simulink model "LQR_observer_R2018a"  (R2018b)
settings: Solver=ode45  StartTime=0.0  StopTime=simulation_time  MaxStep=0.01  RelTol=1e-3  EnableMultiTasking=on
values from neighbouring files (symbols this model uses):
  Cprime = sol2.getCprime    [exercise2_LQRandObserver.m]
  L = parameters(2)    [ex1.m]    (also in exercise2_LQRandObserver.m = L_options{exp_id})
  noiseMod = sol2.getNoiseModule    [exercise2_LQRandObserver.m]
  path_to_track = []    [exercise3_DynamicProgramming.m]
  Phi = Md.A    [ex1.m]
  sampling_time = 0.1    [exercise1_Linearization.m]    (also in exercise2_LQRandObserver.m = 0.005; exercise3_DynamicProgramming.m = 0.24)
  x0 = {x0_experiment_1,                  x0_experiment_1,                  x0_experiment_1,                  x0_experiment_1,                  x0_experiment_1}    [ex1.m]    (also in ex3.m = [0, 0, 0, 0, 0]'; exercise1_Linearization.m = x0_experiments{exp_id}; exercise3_DynamicProgramming.m = sol3.getInitialState)
undefined symbols (not defined in the file or in its folder): CMes, CObs, DObs, Gam, KDlqr, x0Obs
settings Model: Creator=ezequiel  LastModifiedBy=arne
settings OptimizationCC: LifeSpan=inf
settings DebuggingCC: AllowSymbolicDim=off  LibraryContextMissingDiagnostic=none  SFUnexpectedBacktrackingDiag=warning  SFNoUnconditionalDefaultTransitionDiag=warning  SFExecutionAtInitializationDiag=none
settings ModelReferenceCC: PropagateSignalLabelsOutOfModel=off
settings SFSimCC: SimUseLocalCustomCode=off
settings RTWCC: RTWUseLocalCustomCode=off
settings CodeAppCC: StateflowObjectComments=on
settings GRTTargetCC: TargetLangStandard=C89/C90 (ANSI)
settings ConfigComp: CovMetricSettings=dw  CovHtmlReporting=on  CovSaveCumulativeToWorkspaceVar=on  CovSaveSingleToWorkspaceVar=on  CovExternalEMLEnable=off

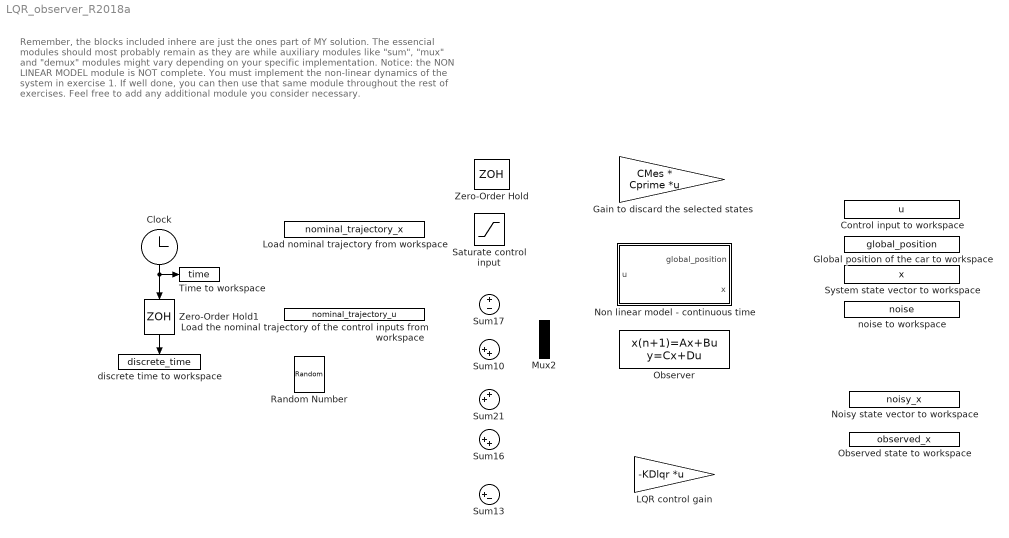
== system LQR_observer_R2018a ==
  note: Remember, the blocks included inhere are just the ones part of MY solution. The essencial modules should most probably remain as they are while auxiliary modules like "sum", "mux" and "demux" modules might vary depending on your specific implementation.
      |
      | Notice: the NON LINEAR MODEL module is NOT complete. You must implement the non-linear dynamics of the system in exercise 1. If well done, you can then use that same module throughout the rest of exercises.
      |
      | Feel free to add any additional module you consider necessary.
  Clock : Clock
  Control input to workspace : ToWorkspace  VariableName=u  SampleTime=-1
  Gain to discard the selected states : Gain  Gain=CMes * Cprime  Multiplication=Matrix(K*u)  SampleTime=sampling_time
  Global position of the car to workspace : ToWorkspace  VariableName=global_position  SampleTime=-1
  LQR control gain : Gain  Gain=-KDlqr  Multiplication=Matrix(K*u)  SampleTime=sampling_time
  Load nominal trajectory from workspace : FromWorkspace  VariableName=nominal_trajectory_x  SampleTime=sampling_time  Interpolate=off  OutputAfterFinalValue=Holding final value
  Load the nominal trajectory of the control inputs from workspace : FromWorkspace  VariableName=nominal_trajectory_u  SampleTime=sampling_time  Interpolate=off  OutputAfterFinalValue=Holding final value
  Mux2 : Mux  Inputs=2
  Noisy state vector to workspace : ToWorkspace  VariableName=noisy_x  SampleTime=-1
  Non linear model - continuous time : Subsystem
  Observed state to workspace : ToWorkspace  VariableName=observed_x  SampleTime=-1
  Observer : DiscreteStateSpace  A=Phi-L*CMes  B=[Gam L]  C=CObs  D=DObs  InitialCondition=x0Obs  SampleTime=sampling_time
  Random Number : RandomNumber  Mean=noiseMod.mean  Variance=noiseMod.std_deviation.^2  Seed=noiseMod.seed  SampleTime=sampling_time
  Saturate control input : Saturate  UpperLimit=[Inf;pi/4]  LowerLimit=[0;-pi/4]
  Sum10 : Sum  Inputs=|++
  Sum13 : Sum  Inputs=|+-
  Sum16 : Sum  Inputs=|++
  Sum17 : Sum  Inputs=+|-
  Sum21 : Sum  Inputs=++|
  System state vector to workspace : ToWorkspace  VariableName=x  SampleTime=-1
  Time to workspace : ToWorkspace  VariableName=time  SampleTime=-1
  Zero-Order Hold : ZeroOrderHold  SampleTime=sampling_time
  Zero-Order Hold1 : ZeroOrderHold  SampleTime=sampling_time
  discrete time to workspace : ToWorkspace  VariableName=discrete_time  SampleTime=-1
  noise to workspace : ToWorkspace  VariableName=noise  SampleTime=-1
  wires:
  Zero-Order Hold1/1 -> discrete time to workspace/1
  Clock/1 -> Zero-Order Hold1/1, Time to workspace/1

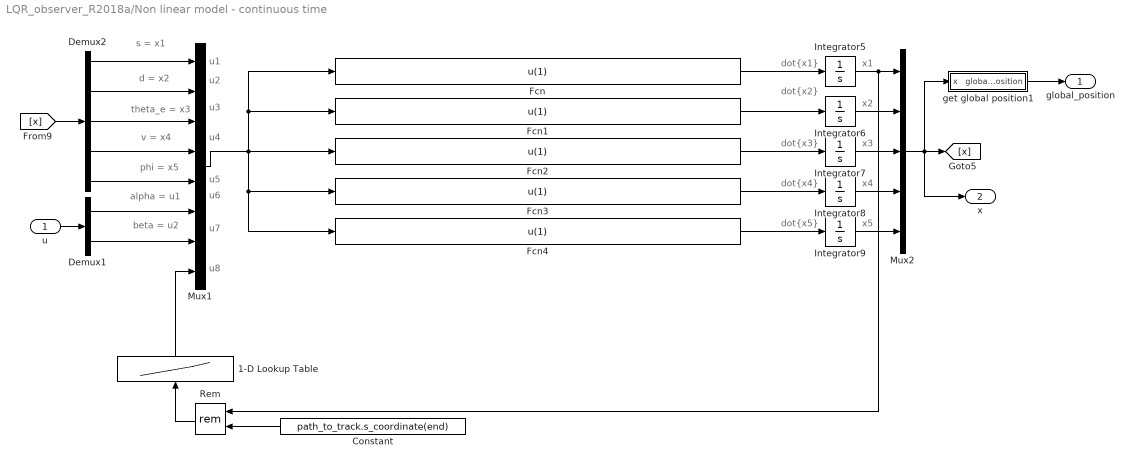
== system LQR_observer_R2018a/Non linear model - continuous time ==
  note: s = x1
  note: dot{x1}
  note: d = x2
  note: theta_e = x3
  note: v = x4
  note: phi = x5
  note: alpha = u1
  note: beta = u2
  note: u1
  note: u2
  note: u3
  note: u4
  note: u5
  note: u6
  note: u7
  note: x1
  note: dot{x2}
  note: x2
  note: dot{x3}
  note: x3
  note: dot{x4}
  note: x4
  note: dot{x5}
  note: x5
  note: u8
  u : Inport
  1-D Lookup Table : Lookup_n-D  NumberOfTableDimensions=1  BreakpointsForDimension1=path_to_track.s_coordinate  Table=path_to_track.curvature  InternalRulePriority=Speed  RndMeth=Simplest  InputSameDT=on
  Constant : Constant  Value=path_to_track.s_coordinate(end)
  Demux1 : Demux  Outputs=2
  Demux2 : Demux  Outputs=5
  Fcn{,1..4} (5 alike) : Fcn  Expr=u(1)
  Integrator5 : Integrator  InitialCondition=x0(1)
  Integrator6 : Integrator  InitialCondition=x0(2)
  Integrator7 : Integrator  InitialCondition=x0(3)
  Integrator8 : Integrator  InitialCondition=x0(4)
  Integrator9 : Integrator  InitialCondition=x0(5)
  Mux1 : Mux  Inputs=8
  Mux2 : Mux  Inputs=5
  Rem : Math  Operator=rem  SaturateOnIntegerOverflow=on
  get global position1 : Subsystem
  global_position : Outport
  x : Outport  Port=2
  wires:
  u/1 -> Demux1/1
  Fcn/1 -> Integrator5/1
  Demux2/1 -> Mux1/1
  Demux2/2 -> Mux1/2
  Demux2/3 -> Mux1/3
  Demux2/4 -> Mux1/4
  Demux2/5 -> Mux1/5
  Demux1/1 -> Mux1/6
  Demux1/2 -> Mux1/7
  Mux1/1 -> Fcn3/1, Fcn4/1, Fcn1/1, Fcn/1, Fcn2/1
  Fcn1/1 -> Integrator6/1
  Integrator6/1 -> Mux2/2
  Fcn2/1 -> Integrator7/1
  Integrator7/1 -> Mux2/3
  Fcn3/1 -> Integrator8/1
  Integrator8/1 -> Mux2/4
  Fcn4/1 -> Integrator9/1
  Integrator9/1 -> Mux2/5
  [x] -> Demux2/1
  1-D Lookup Table/1 -> Mux1/8
  Rem/1 -> 1-D Lookup Table/1
  Constant/1 -> Rem/2
  Integrator5/1 -> Rem/1, Mux2/1
  Mux2/1 -> get global position1/1(x), x/1, [x]
  get global position1/1(global_position) -> global_position/1

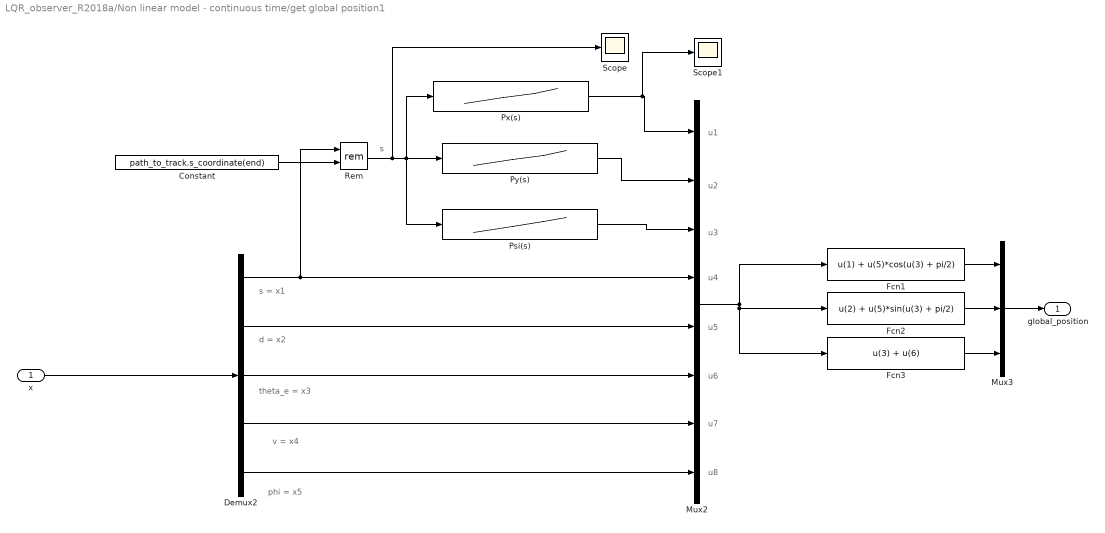
== system LQR_observer_R2018a/Non linear model - continuous time/get global position1 ==
  note: s
  note: s = x1
  note: d = x2
  note: theta_e = x3
  note: v = x4
  note: phi = x5
  note: u1
  note: u2
  note: u3
  note: u4
  note: u5
  note: u6
  note: u7
  note: u8
  x : Inport
  Constant : Constant  Value=path_to_track.s_coordinate(end)
  Demux2 : Demux  Outputs=5
  Fcn1 : Fcn  Expr=u(1) + u(5)*cos(u(3) + pi/2)
  Fcn2 : Fcn  Expr=u(2) + u(5)*sin(u(3) + pi/2)
  Fcn3 : Fcn  Expr=u(3) + u(6)
  Mux2 : Mux  Inputs=8
  Mux3 : Mux  Inputs=3
  Psi(s) : Lookup_n-D  NumberOfTableDimensions=1  BreakpointsForDimension1=path_to_track.s_coordinate  Table=path_to_track.orientation  InternalRulePriority=Speed  RndMeth=Simplest  InputSameDT=on
  Px(s) : Lookup_n-D  NumberOfTableDimensions=1  BreakpointsForDimension1=path_to_track.s_coordinate  Table=path_to_track.coordinates(:,1)  InternalRulePriority=Speed  RndMeth=Simplest  InputSameDT=on
  Py(s) : Lookup_n-D  NumberOfTableDimensions=1  BreakpointsForDimension1=path_to_track.s_coordinate  Table=path_to_track.coordinates(:,2)  InternalRulePriority=Speed  RndMeth=Simplest  InputSameDT=on
  Rem : Math  Operator=rem  SaturateOnIntegerOverflow=on
  Scope : Scope
  Scope1 : Scope
  global_position : Outport
  wires:
  Demux2/1 -> Mux2/4, Rem/1
  Mux3/1 -> global_position/1
  x/1 -> Demux2/1
  Rem/1 -> Scope/1, Psi(s)/1, Px(s)/1, Py(s)/1
  Constant/1 -> Rem/2
  Px(s)/1 -> Scope1/1, Mux2/1
  Py(s)/1 -> Mux2/2
  Psi(s)/1 -> Mux2/3
  Mux2/1 -> Fcn3/1, Fcn2/1, Fcn1/1
  Fcn1/1 -> Mux3/1
  Fcn2/1 -> Mux3/2
  Fcn3/1 -> Mux3/3
  Demux2/2 -> Mux2/5
  Demux2/3 -> Mux2/6
  Demux2/4 -> Mux2/7
  Demux2/5 -> Mux2/8
